simulink model "DCACDC"  (R2018b)
settings: Solver=ode23  StartTime=0.0  StopTime=0.05  MaxStep=1e-4  RelTol=1e-3
values from neighbouring files (symbols this model uses):
  C = 470e-6    (= 0.00047)    [Parameter_DAD.m]    (also in Parameter_PFC.m = 7.2e-10)
  C_oss = 270e-12    (= 2.7e-10)    [Parameter_DAD.m]
  Cr = 66e-9    (= 6.6e-08)    [Parameter_DAD.m]
  I_u = 10    [Parameter_DAD.m]    (also in Parameter_PFC.m)
  L = 50*1e-4    (= 0.005)    [Parameter_DAD.m]    (also in Parameter_PFC.m = 0.003)
  Lm = 100e-6    (= 0.0001)    [Parameter_DAD.m]
  Lr = 10e-6    (= 1e-05)    [Parameter_DAD.m]
  n = floor(400/48)    [Parameter_DAD.m]
  P_u = 5    [Parameter_DAD.m]    (also in Parameter_PFC.m = 0.1)
  R_load = V_out*V_out/ratio/P    (= 7.2)    [Parameter_DAD.m]
  U_trgt = 48    [Parameter_DAD.m]
  V_in = 400    [Parameter_DAD.m]    (also in Parameter_PFC.m = 31.108)
libraries: powerlib x30, powerlib_meascontrol x2, simulink x1
settings Model: Creator=lenovo  LastModifiedBy=lenovo
settings DebuggingCC: MaxConsecutiveZCsMsg=none
settings SFSimCC: SimUseLocalCustomCode=off
settings RTWCC: RTWUseLocalCustomCode=off
settings CodeAppCC: StateflowObjectComments=on
settings SimscapeCC: SimscapeNormalizeSystem=off

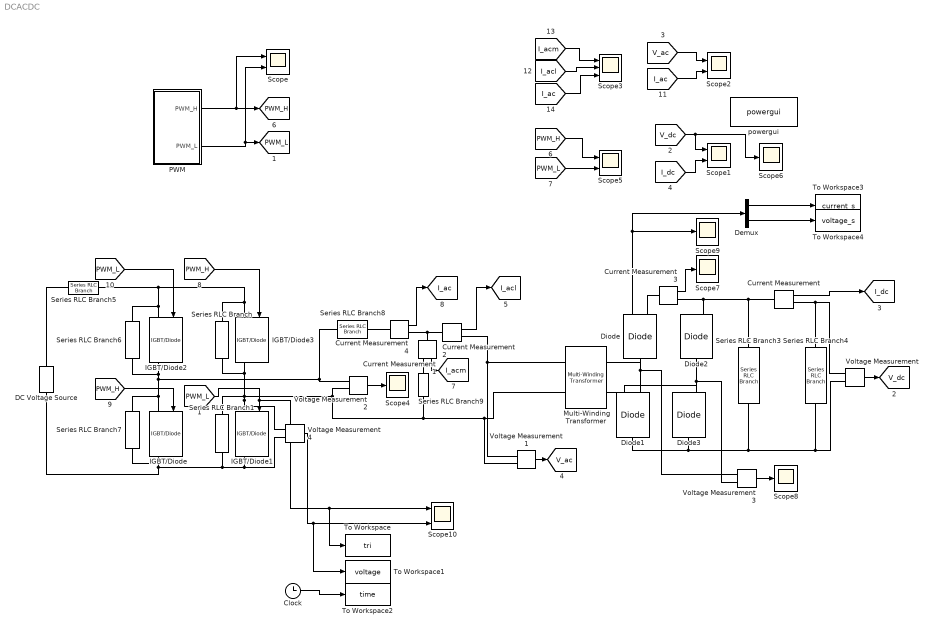
== system DCACDC ==
  Clock : Clock
  Current Measurement{,1..4} (5 alike) : powerlib/Measurements/Current Measurement  PhasorSimulation=off  OutputType=Complex  PSBequivalent=0
      settings: SourceProductName=Simscape Electrical
  DC Voltage Source : powerlib/Electrical Sources/DC Voltage Source  Amplitude=V_in  Measurements=None
      settings: SourceProductName=Simscape Electrical
  Demux : Demux  Outputs=2
  Diode{,1..3} (4 alike) : powerlib/Power Electronics/Diode  Ron=0.001  Lon=0  Vf=0.8  IC=0  UseSnubber=0  Rs=500  Cs=250e-9  Measurements=on
      settings: SourceProductName=Simscape Electrical
  IGBT/Diode{,1..3} (4 alike) : powerlib/Power Electronics/IGBT//Diode  Ron=1e-3  Rs=1e5  Cs=inf  Measurements=on
  Multi-Winding Transformer : powerlib/Elements/Multi-Winding Transformer  LeftWindings=1  RightWindings=1  TappedWindings=no taps  NumberOfTaps=2  SetSaturation=off  Hysteresis=off  DataFile='hysteresis.mat'  Measurements=None  UNITS=pu  NominalPower=[500 5e5]  NominalVoltages="[ 400  400/n]"  WindingResistances="[ 0.005  0.005]"  WindingInductances="[ 0.02  0.02 ]"  Rm=50  Lm=50  Saturation=[ 0,0 ; 0.0024,1.2 ; 1.0,1.52 ]  MoreParameters=off  BreakLoop=off  DataType=off  InitialFlux=0  TransfoNumber=1
      settings: SourceProductName=Simscape Power Systems  SourceProductBaseCode=PS
  PWM : Subsystem
  Scope{,1..2,5,10} (5 alike) : Scope  NumInputPorts=2
  Scope3 : Scope  NumInputPorts=3
  Scope{4,6..9} (5 alike) : Scope
  Series RLC Branch{,1,6..7} (4 alike) : powerlib/Elements/Series RLC Branch  LConnTagsString=__new0  RConnTagsString=__new0  BranchType=C  Resistance=1  Inductance=1e-3  SetiL0=off  InitialCurrent=0  Capacitance=C_oss  Setx0=off  InitialVoltage=V_in/2  Measurements=None
      settings: SourceProductName=Simscape Electrical
  Series RLC Branch3 : powerlib/Elements/Series RLC Branch  LConnTagsString=__new0  RConnTagsString=__new0  BranchType=C  Resistance=1  Inductance=1e-3  SetiL0=off  InitialCurrent=0  Capacitance=C  Setx0=off  InitialVoltage=0  Measurements=None
      settings: SourceProductName=Simscape Electrical
  Series RLC Branch4 : powerlib/Elements/Series RLC Branch  LConnTagsString=__new0  RConnTagsString=__new0  BranchType=R  Resistance=R_load  Inductance=1e-3  SetiL0=off  InitialCurrent=0  Capacitance=C  Setx0=off  InitialVoltage=0  Measurements=None
      settings: SourceProductName=Simscape Electrical
  Series RLC Branch5 : powerlib/Elements/Series RLC Branch  LConnTagsString=__new0  RConnTagsString=__new0  BranchType=R  Resistance=1e-3  Inductance=L  SetiL0=off  InitialCurrent=0  Capacitance=C  Setx0=off  InitialVoltage=0  Measurements=None
      settings: SourceProductName=Simscape Electrical
  Series RLC Branch8 : powerlib/Elements/Series RLC Branch  LConnTagsString=__new0  RConnTagsString=__new0  BranchType=LC  Resistance=1  Inductance=Lr  SetiL0=off  InitialCurrent=0  Capacitance=Cr  Setx0=off  InitialVoltage=0  Measurements=None
      settings: SourceProductName=Simscape Electrical
  Series RLC Branch9 : powerlib/Elements/Series RLC Branch  LConnTagsString=__new0  RConnTagsString=__new0  BranchType=L  Resistance=1  Inductance=Lm  SetiL0=off  InitialCurrent=0  Capacitance=C  Setx0=off  InitialVoltage=0  Measurements=None
      settings: SourceProductName=Simscape Electrical
  To Workspace : ToWorkspace  VariableName=tri  SaveFormat=Timeseries  SampleTime=-1
  To Workspace1 : ToWorkspace  VariableName=voltage  SaveFormat=Timeseries  SampleTime=-1
  To Workspace2 : ToWorkspace  VariableName=time  SaveFormat=Timeseries  SampleTime=-1
  To Workspace3 : ToWorkspace  VariableName=current_s  SaveFormat=Timeseries  SampleTime=-1
  To Workspace4 : ToWorkspace  VariableName=voltage_s  SaveFormat=Timeseries  SampleTime=-1
  Voltage Measurement{,1..4} (5 alike) : powerlib/Measurements/Voltage Measurement  PhasorSimulation=off  OutputType=Complex  PSBequivalent=0
      settings: SourceProductName=Simscape Electrical
  powergui : powerlib/powergui  SimulationMode=Discrete  SampleTime=1e-8  frequency=60  Iterations=50  frequencyindice=0  Pbase=100e6  ErrMax=1e-4  UnitsV=kV  UnitsW=MW  buscounter=0  FunctionMessages=off  echomessages=off  EnableUseOfTLC=off  CurrentSourceSwitches=off  DisableSnubberDevices=off  DisableRonSwitches=off  DisableVfSwitches=off  DisplayEquations=off  SolverType=Tustin/Backward Euler (TBE)  Interpol=off  ExternalGateDelay=off  methode=off  Ts=100  x0status=blocks  SPID=off  SwTol=0  HookPort=off  RestoreLinks=warning  ResistiveCurrentMeasurement=off  Frange=[0:2:500]  Ylog=off  Xlog=on  ShowGrid=off  save=off  variable=ZData  structure=ScopeData2  ZoomFFT=off  StartTime=0.7  cycles=10  DisplayStyle=1  fundamental=50  FreqAxis=off  MaxFrequency=12000  frequencyindicesteady=1  RmsSteady=1  display=off
  tag scope: I_ac=global, I_acl=global, I_acm=global, I_dc=global, PWM_H=global, PWM_L=global, V_ac=global, V_dc=global
  wires:
  PWM/1(PWM_H) -> Scope/1, [PWM_H]
  PWM/2(PWM_L) -> Scope/2, [PWM_L]
  [V_dc] -> Scope1/1, Scope6/1
  [I_dc] -> Scope1/2
  [V_ac] -> Scope2/1
  [PWM_H] -> Scope5/1
  [PWM_L] -> Scope5/2
  [I_ac] -> Scope2/2
  [I_acl] -> Scope3/2
  [I_acm] -> Scope3/1
  [I_ac] -> Scope3/3
  Voltage Measurement/1 -> [V_dc]
  Voltage Measurement3/1 -> Scope8/1
  Current Measurement4/1 -> [I_ac]
  Current Measurement/1 -> [I_dc]
  Current Measurement2/1 -> [I_acl]
  Voltage Measurement2/1 -> Scope4/1
  Current Measurement1/1 -> [I_acm]
  [PWM_L] -> IGBT/Diode2/1
  [PWM_L] -> To Workspace/1, Scope10/1, IGBT/Diode1/1
  [PWM_H] -> IGBT/Diode/1
  Voltage Measurement1/1 -> [V_ac]
  [PWM_H] -> IGBT/Diode3/1
  Current Measurement3/1 -> Scope7/1
  Diode/1 -> Demux/1, Scope9/1
  Voltage Measurement4/1 -> To Workspace1/1, Scope10/2
  Clock/1 -> To Workspace2/1
  Demux/1 -> To Workspace3/1
  Demux/2 -> To Workspace4/1
  connections:
  Diode1/LConn1 -- Diode3/LConn1 -- Series RLC Branch3/RConn1 -- Voltage Measurement/LConn2 -- Series RLC Branch4/RConn1
  Voltage Measurement2/LConn2 -- Voltage Measurement4/LConn1 -- IGBT/Diode1/LConn1 -- Series RLC Branch1/LConn1 -- IGBT/Diode3/RConn1 -- Series RLC Branch/RConn1 -- Multi-Winding Transformer/LConn2 -- Voltage Measurement1/LConn2 -- Series RLC Branch9/LConn1
  Multi-Winding Transformer/LConn1 -- Current Measurement2/RConn1 -- Voltage Measurement1/LConn1
  Series RLC Branch3/LConn1 -- Diode2/RConn1 -- Current Measurement3/RConn1 -- Current Measurement/LConn1
  Voltage Measurement3/LConn1 -- Diode1/RConn1 -- Multi-Winding Transformer/RConn1 -- Diode/LConn1
  Current Measurement4/RConn1 -- Current Measurement2/LConn1 -- Current Measurement1/LConn1
  Current Measurement/RConn1 -- Series RLC Branch4/LConn1 -- Voltage Measurement/LConn1
  Series RLC Branch6/RConn1 -- IGBT/Diode2/RConn1 -- Voltage Measurement2/LConn1 -- Series RLC Branch8/RConn1 -- Series RLC Branch7/LConn1 -- IGBT/Diode/LConn1
  Diode2/LConn1 -- Diode3/RConn1 -- Multi-Winding Transformer/RConn2 -- Voltage Measurement3/LConn2
  Series RLC Branch/LConn1 -- Series RLC Branch5/LConn1 -- IGBT/Diode2/LConn1 -- Series RLC Branch6/LConn1 -- IGBT/Diode3/LConn1
  Current Measurement1/RConn1 -- Series RLC Branch9/RConn1
  Current Measurement4/LConn1 -- Series RLC Branch8/LConn1
  Series RLC Branch5/RConn1 -- DC Voltage Source/RConn1
  Current Measurement3/LConn1 -- Diode/RConn1
  IGBT/Diode1/RConn1 -- DC Voltage Source/LConn1 -- Series RLC Branch7/RConn1 -- IGBT/Diode/RConn1 -- Series RLC Branch1/RConn1 -- Voltage Measurement4/LConn2

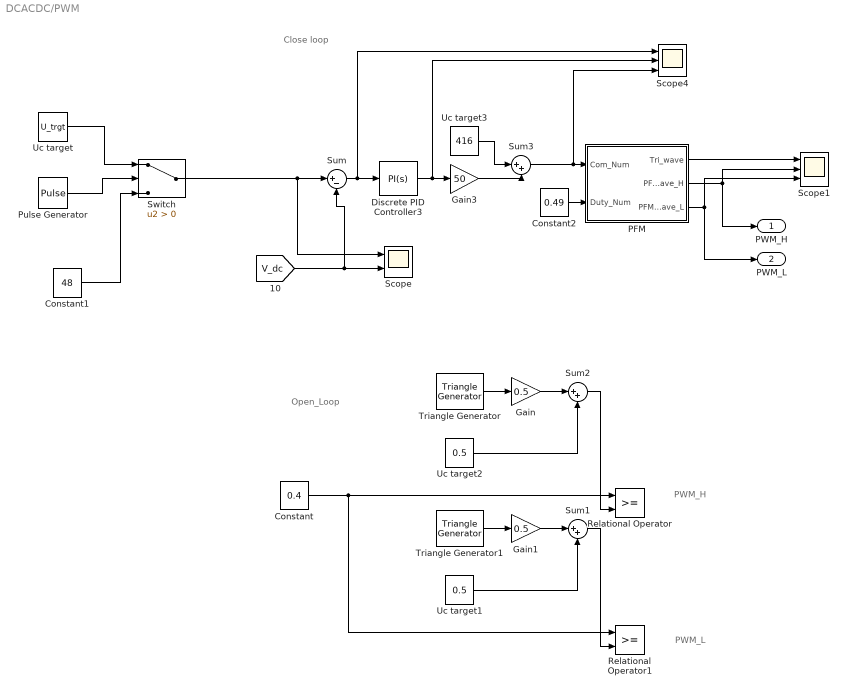
== system DCACDC/PWM ==
  note: Close loop
  note: Open_Loop
  note: PWM_L
  note: PWM_H
  Constant : Constant  Value=0.4
  Constant1 : Constant  Value=48
  Constant2 : Constant  Value=0.49
  Discrete PID Controller3 : simulink/Continuous/PID Controller  Controller=PI  Form=Parallel  TimeDomain=Continuous-time  SampleTime=-1  IntegratorMethod=Forward Euler  FilterMethod=Forward Euler  ControllerParametersSource=internal  P=P_u  I=I_u  D=0  UseFilter=on  N=100  TunerSelectOption=Transfer Function Based (PID Tuner App)  InitialConditionSource=internal  InitialConditionForIntegrator=0  InitialConditionForFilter=0  DifferentiatorICPrevScaledInput=0  ExternalReset=none  TrackingMode=off  Kt=1  LimitOutput=on  UpperSaturationLimit=5  LowerSaturationLimit=-10  LinearizeAsGain=off  AntiWindupMode=none  Kb=1  POutMin=[]  POutMax=[]  IOutMin=[]  IOutMax=[]  DOutMin=[]  DOutMax=[]  NOutMin=[]  NOutMax=[]  SumOutMin=[]  SumOutMax=[]  SaturationOutMin=[]  SaturationOutMax=[]  PParamMin=[]  PParamMax=[]  IParamMin=[]  IParamMax=[]  DParamMin=[]  DParamMax=[]  NParamMin=[]  NParamMax=[]  KbParamMin=[]  KbParamMax=[]  KtParamMin=[]  KtParamMax=[]  KbOutMin=[]  KbOutMax=[]  KtOutMin=[]  KtOutMax=[]  IntegratorOutMin=[]  IntegratorOutMax=[]  FilterOutMin=[]  FilterOutMax=[]  SumI1OutMin=[]  SumI1OutMax=[]  SumI2OutMin=[]  SumI2OutMax=[]  SumI3OutMin=[]  SumI3OutMax=[]  SumI4OutMin=[]  SumI4OutMax=[]  SumDOutMin=[]  SumDOutMax=[]  DifferentiatorOutMin=[]  DifferentiatorOutMax=[]  FilterDiffOutCoefMin=[]  FilterDiffOutCoefMax=[]  ReciprocalOutMin=[]  ReciprocalOutMax=[]  SumDenOutMin=[]  SumDenOutMax=[]  SumNumOutMin=[]  SumNumOutMax=[]  DivideOutMin=[]  DivideOutMax=[]  IntegratorContinuousStateAttributes=''  IntegratorStateMustResolveToSignalObject=off  IntegratorRTWStateStorageClass=Auto  FilterContinuousStateAttributes=''  FilterStateMustResolveToSignalObject=off  FilterRTWStateStorageClass=Auto  ParallelPVariant=InternalParameters  IdealPVariant=Disabled  IVariant=InternalParameters  DVariant=Disabled  IntegratorVariant=Continuous  SatVariant=Enabled  AWVariant=Passthrough  PCopyVariant=Disabled  TRVariant=Disabled  FdbkBlocksVariant=Forward  IdealPFdbkVariant=Disabled  SatFdbkVariant=Disabled  DerivativeFilterVariant=Disabled  NVariant=Disabled  NCopyVariant=Disabled_SignalSpec  FilterICVariant=Disabled  IntegratorICVariant=InternalICs  ExternalResetVariant=Disabled  TRSumVariant=Passthrough  SumFdbkVariant=Disabled  SumVariant=Sum_PI
  Gain : Gain  Gain=0.5
  Gain1 : Gain  Gain=0.5
  Gain3 : Gain  Gain=50
  PFM : Subsystem
  Pulse Generator : DiscretePulseGenerator  PulseType=Time based  Period=0.005  PulseWidth=50
  Relational Operator : RelationalOperator  OutDataTypeStr=boolean  RndMeth=Simplest
  Relational Operator1 : RelationalOperator  OutDataTypeStr=boolean  RndMeth=Simplest
  Scope : Scope  NumInputPorts=2
  Scope1 : Scope  NumInputPorts=3
  Scope4 : Scope  NumInputPorts=3
  Sum : Sum  Inputs=|+-
  Sum1 : Sum  Inputs=|++
  Sum2 : Sum  Inputs=|++
  Sum3 : Sum  Inputs=|++
  Switch : Switch  Criteria=u2 > Threshold
  Triangle Generator : powerlib_meascontrol/Pulse & Signal Generators/Triangle Generator  Freq=f  Phase=90  Ts=0
      settings: SourceProductName=Simscape Electrical
  Triangle Generator1 : powerlib_meascontrol/Pulse & Signal Generators/Triangle Generator  Freq=f  Phase=270  Ts=0
      settings: SourceProductName=Simscape Electrical
  Uc target : Constant  Value=U_trgt
  Uc target1 : Constant  Value=0.5
  Uc target2 : Constant  Value=0.5
  Uc target3 : Constant  Value=416
  PWM_H : Outport
  PWM_L : Outport  Port=2
  wires:
  Sum2/1 -> Relational Operator/2
  Uc target2/1 -> Sum2/2
  Gain/1 -> Sum2/1
  Triangle Generator/1 -> Gain/1
  Sum1/1 -> Relational Operator1/2
  Uc target1/1 -> Sum1/2
  Triangle Generator1/1 -> Gain1/1
  Gain1/1 -> Sum1/1
  Gain3/1 -> Sum3/2
  Discrete PID Controller3/1 -> Scope4/2, Gain3/1
  Sum/1 -> Scope4/1, Discrete PID Controller3/1
  Constant/1 -> Relational Operator1/1, Relational Operator/1
  Constant2/1 -> PFM/2(Duty_Num)
  Uc target3/1 -> Sum3/1
  Sum3/1 -> PFM/1(Com_Num), Scope4/3
  PFM/2(PFM_wave_H) -> Scope1/2, PWM_H/1
  PFM/3(PFM_wave_L) -> Scope1/3, PWM_L/1
  PFM/1(Tri_wave) -> Scope1/1
  Pulse Generator/1 -> Switch/2
  Constant1/1 -> Switch/3
  [V_dc] -> Sum/2, Scope/2
  Uc target/1 -> Switch/1
  Switch/1 -> Scope/1, Sum/1

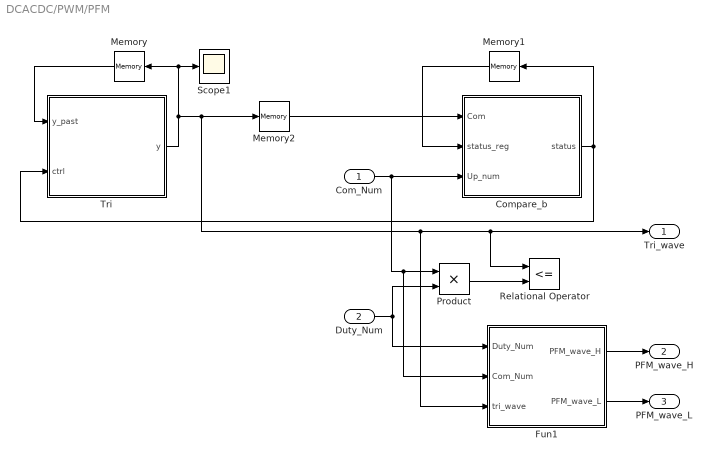
== system DCACDC/PWM/PFM ==
  Com_Num : Inport
  Duty_Num : Inport  Port=2
  Compare_b : MATLAB Function  TreatAsAtomicUnit=on
  Fun1 : MATLAB Function  TreatAsAtomicUnit=on
  Memory : Memory
  Memory1 : Memory
  Memory2 : Memory
  Product : Product
  Relational Operator : RelationalOperator  Operator=<=  OutDataTypeStr=boolean  RndMeth=Simplest
  Scope1 : Scope
  Tri : MATLAB Function  TreatAsAtomicUnit=on
  Tri_wave : Outport
  PFM_wave_H : Outport  Port=2
  PFM_wave_L : Outport  Port=3
  wires:
  Memory1/1 -> Compare_b/2(status_reg)
  Memory/1 -> Tri/1(y_past)
  Com_Num/1 -> Fun1/2(Com_Num), Product/1, Compare_b/3(Up_num)
  Tri/1(y) -> Fun1/3(tri_wave), Relational Operator/1, Tri_wave/1, Memory2/1, Scope1/1, Memory/1
  Memory2/1 -> Compare_b/1(Com)
  Compare_b/1(status) -> Tri/2(ctrl), Memory1/1
  Duty_Num/1 -> Fun1/1(Duty_Num), Product/2
  Product/1 -> Relational Operator/2
  Fun1/1(PFM_wave_H) -> PFM_wave_H/1
  Fun1/2(PFM_wave_L) -> PFM_wave_L/1

== matlab function DCACDC/PWM/PFM/Tri ==
  data: y output; y_past input; ctrl input
function y  = Tri(y_past, ctrl)
if ctrl == 1
    y = y_past + 1;
elseif ctrl == 0
    y = y_past - 1;
else
    y = y_past;
end
end

== matlab function DCACDC/PWM/PFM/Compare_b ==
  data: status output; Com input; status_reg input; Up_num input
function status  = Tri(Com, status_reg, Up_num)
if Com > Up_num
    status = 0;
elseif Com < 0
    status = 1;
else 
    status = status_reg;
end

== matlab function DCACDC/PWM/PFM/Fun1 ==
  data: PFM_wave_H output; Duty_Num input; Com_Num input; tri_wave input; PFM_wave_L output
function [PFM_wave_H,PFM_wave_L] = Tri(Duty_Num, Com_Num, tri_wave)
PFM_wave_H = (tri_wave)<=(Duty_Num*Com_Num);
PFM_wave_L = (tri_wave)>=((1-Duty_Num)*Com_Num);
end
